simulink model "Copy_of_SbW_can_Add"  (R2023b)
settings: Solver=VariableStepAuto  StartTime=0.0  StopTime=20  RelTol=1e-3
model workspace (MAT data in the model file):
  x = 4
undefined symbols (not defined in the file): canChannel
libraries: simulink x5, canlib x3, canmsglib x2
settings Model: Creator=jcm52  LastModifiedBy=jcm52

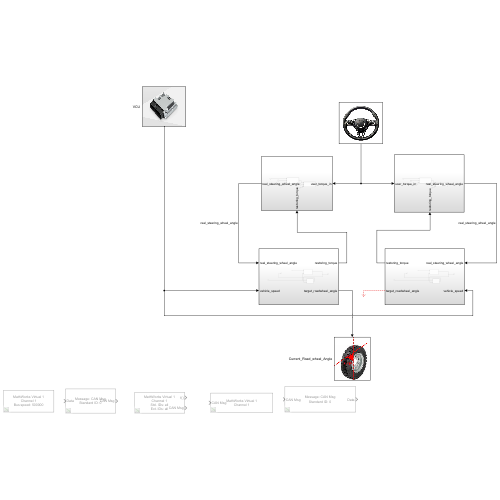
[thumbnail: Simulink's stored preview of the top-level diagram]
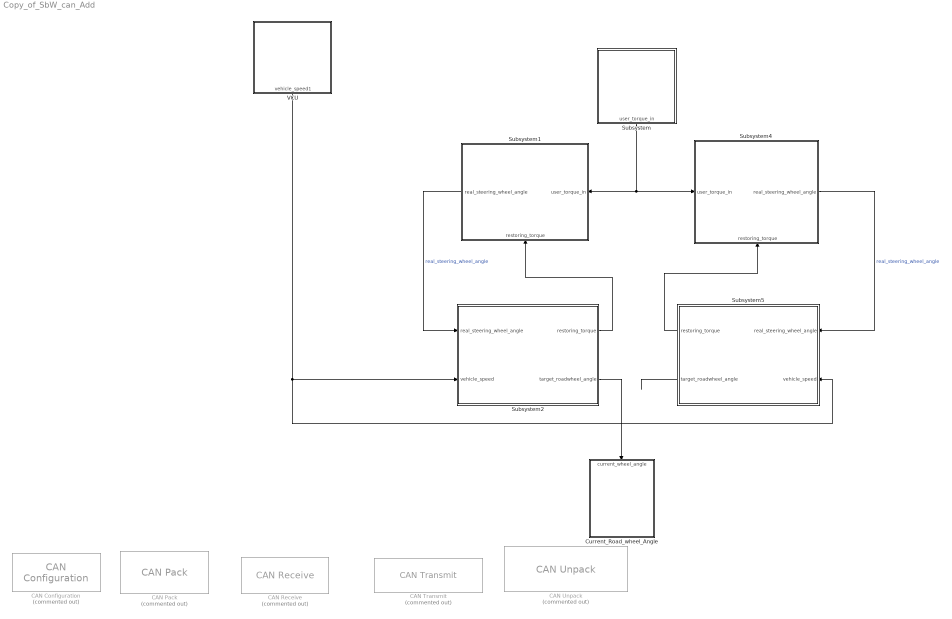
== system Copy_of_SbW_can_Add ==
  CAN Configuration : canlib/CAN Configuration  Commented=on  BlockHandle=2.0012  Device=MathWorks Virtual 1 (Channel 1)  DeviceMenu=MathWorks Virtual 1 (Channel 1)  ObjConstructor=canChannel('MathWorks', 'Virtual 1', 1)  BusSpeed=500000  EnableBitParameters=off  AckMode=Normal
  CAN Pack : canmsglib/CAN Pack  Commented=on  MsgList=(none)  MsgName=CAN Msg  MsgIDType=Standard (11-bit identifier)  MsgIdentifier=0  MsgLength=8  Remote=off  ApplyMinMax=off  BusOutput=off  SignalInfo={}
      settings: LibrarySourceBlock=canlib/CAN Pack  DataFormat=raw data
  CAN Receive : canlib/CAN Receive  Commented=on  BlockHandle=4.0002  Device=MathWorks Virtual 1 (Channel 1)  DeviceMenu=MathWorks Virtual 1 (Channel 1)  ObjConstructor=canChannel('MathWorks', 'Virtual 1', 1)  EnableStandardIDsFilter=off  StdIDsCombo=Allow all  StandardIDs=0  EnableExtendedIDsFilter=off  ExtIDsCombo=Allow all  ExtendedIDs=0  SampleTime=0.01  MsgsPerTimestep=all  InternalFilterUpdateStatus=on  BusOutput=off
  CAN Transmit : canlib/CAN Transmit  Commented=on  BlockHandle=5.0002  Device=MathWorks Virtual 1 (Channel 1)  DeviceMenu=MathWorks Virtual 1 (Channel 1)  ObjConstructor=canChannel('MathWorks', 'Virtual 1', 1)  EnableEventTransmit=off  EnablePeriodicTransmit=off  MessagePeriod=1.000
  CAN Unpack : canmsglib/CAN Unpack  Commented=on  MsgList=(none)  MsgName=CAN Msg  MsgIDType=Standard (11-bit identifier)  MsgIdentifier=0  MsgLength=8  SignalInfo={}  IDPort=off  TimestampPort=off  ErrorPort=off  RemotePort=off  LengthPort=off  StatusPort=off  ApplyMinMax=off
      settings: LibrarySourceBlock=canlib/CAN Unpack  DataFormat=raw data
  Current_Road_wheel_Angle : Subsystem
      mask Display: image('image\road_wheel_angle.JPG');
  Subsystem : Subsystem
      mask Display: image('image\pngtree-car-steering-wheel-png-image_13061877.png');
  Subsystem1 : Subsystem
      settings: PortSchema="{\"entries\":[{\"content\":{\"sides\":[{\"content\":{\"connectorIds\":[\"In1\"]},\"type\":\"ConnectorPlacement.EquallySpacedRectSide\",\"uuid\":\"9f784dfa-5041-4500-abe3-8ca3b2947121\"},{\"content\":{\"connectorIds\":[\"Out1\"],\"side\":\"RIGHT\"},\"type\":\"ConnectorPlacement.EquallySpacedRectSide\",\"uuid\":\"b0f943eb-3587-44b5-9c58-09c6c0469d22\"},{\"content\":{\"connectorIds\":[\"In2\"],\"side\":\"TOP\"},\"type\":\"ConnectorPlacement.EquallySpacedRectSide\",\"uuid\":\"b1f972b4-0000-4041-88f3-3b96e8f3d0bc\"},{\"content\":{\"side\":\"BOTTOM\"},\"type\":\"ConnectorPlacement.EquallySpacedRectSide\",\"uuid\":\"3fad1dd4-0e91-4329-9148-3a998504f86d\"}]},\"type\":\"ConnectorPlacement.EquallySpacedConnector\",\"uuid\":\"65662e9c-02e8-4401-a13c-81033cd1290c\"}],\"packageUris\":[\"http://schema.mathworks.com/mf0/Connector/R2020b\"],\"version\":\"1.0\"}"
  Subsystem2 : Subsystem
  Subsystem4 : Subsystem
      settings: PortSchema="{\"entries\":[{\"content\":{\"sides\":[{\"content\":{\"connectorIds\":[\"In1\"]},\"type\":\"ConnectorPlacement.EquallySpacedRectSide\",\"uuid\":\"9f784dfa-5041-4500-abe3-8ca3b2947121\"},{\"content\":{\"connectorIds\":[\"Out1\"],\"side\":\"RIGHT\"},\"type\":\"ConnectorPlacement.EquallySpacedRectSide\",\"uuid\":\"b0f943eb-3587-44b5-9c58-09c6c0469d22\"},{\"content\":{\"side\":\"TOP\"},\"type\":\"ConnectorPlacement.EquallySpacedRectSide\",\"uuid\":\"b1f972b4-0000-4041-88f3-3b96e8f3d0bc\"},{\"content\":{\"connectorIds\":[\"In2\"],\"side\":\"BOTTOM\"},\"type\":\"ConnectorPlacement.EquallySpacedRectSide\",\"uuid\":\"3fad1dd4-0e91-4329-9148-3a998504f86d\"}]},\"type\":\"ConnectorPlacement.EquallySpacedConnector\",\"uuid\":\"65662e9c-02e8-4401-a13c-81033cd1290c\"}],\"packageUris\":[\"http://schema.mathworks.com/mf0/Connector/R2020b\"],\"version\":\"1.0\"}"
  Subsystem5 : Subsystem
  VCU : Subsystem
      mask Display: image('image\vehicle-control-unit-compare-view-01_teaser.jpg');
  wires:
  Subsystem1/1(real_steering_wheel_angle) -> Subsystem2/1(real_steering_wheel_angle)  "real_steering_wheel_angle"
  Subsystem2/1(restoring_torque) -> Subsystem1/2(restoring_torque)
  Subsystem2/2(target_roadwheel_angle) -> Current_Road_wheel_Angle/1(current_wheel_angle)
  Subsystem/1(user_torque_in) -> Subsystem4/1(user_torque_in), Subsystem1/1(user_torque_in)
  Subsystem4/1(real_steering_wheel_angle) -> Subsystem5/1(real_steering_wheel_angle)  "real_steering_wheel_angle"
  Subsystem5/1(restoring_torque) -> Subsystem4/2(restoring_torque)
  VCU/1(vehicle_speed1) -> Subsystem5/2(vehicle_speed), Subsystem2/2(vehicle_speed)
  Subsystem5/2(target_roadwheel_angle) -> ?

== system Copy_of_SbW_can_Add/Current_Road_wheel_Angle ==
  current_wheel_angle : Inport

== system Copy_of_SbW_can_Add/Subsystem ==
  Bias : Bias  Bias=x  SaturateOnIntegerOverflow=off
  pulse_torque_in2 : DiscretePulseGenerator  PulseType=Time based  Amplitude=2*x  Period=5  PulseWidth=50
      mask Display: image('image\pngtree-car-steering-wheel-png-image_13061877.png');
  user_torque_in : Outport
  wires:
  pulse_torque_in2/1 -> Bias/1  "Torque_in"
  Bias/1 -> user_torque_in/1  "user_torque_in"

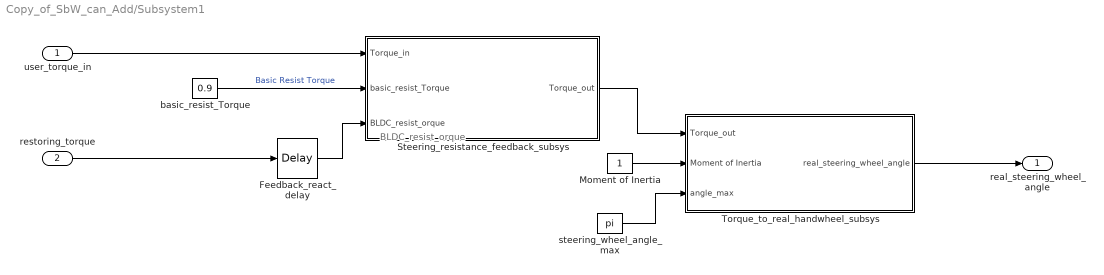
== system Copy_of_SbW_can_Add/Subsystem1 ==
  note: BLDC_resist_orque
  user_torque_in : Inport
  restoring_torque : Inport  Port=2
  Feedback_react_delay : TransportDelay  DelayTime=0.02
  Moment of Inertia : Constant
  Steering_resistance_feedback_subsys : Subsystem
  Torque_to_real_handwheel_subsys : Subsystem
  basic_resist_Torque : Constant  Value=0.9  SampleTime=0.001
  steering_wheel_angle_max : Constant  Value=pi
  real_steering_wheel_angle : Outport
  wires:
  restoring_torque/1 -> Feedback_react_delay/1
  Steering_resistance_feedback_subsys/1(Torque_out) -> Torque_to_real_handwheel_subsys/1(Torque_out)
  steering_wheel_angle_max/1 -> Torque_to_real_handwheel_subsys/3(angle_max)
  Torque_to_real_handwheel_subsys/1(real_steering_wheel_angle) -> real_steering_wheel_angle/1
  Feedback_react_delay/1 -> Steering_resistance_feedback_subsys/3(BLDC_resist_orque)
  Moment of Inertia/1 -> Torque_to_real_handwheel_subsys/2(Moment of Inertia)
  user_torque_in/1 -> Steering_resistance_feedback_subsys/1(Torque_in)
  basic_resist_Torque/1 -> Steering_resistance_feedback_subsys/2(basic_resist_Torque)  "Basic Resist Torque"

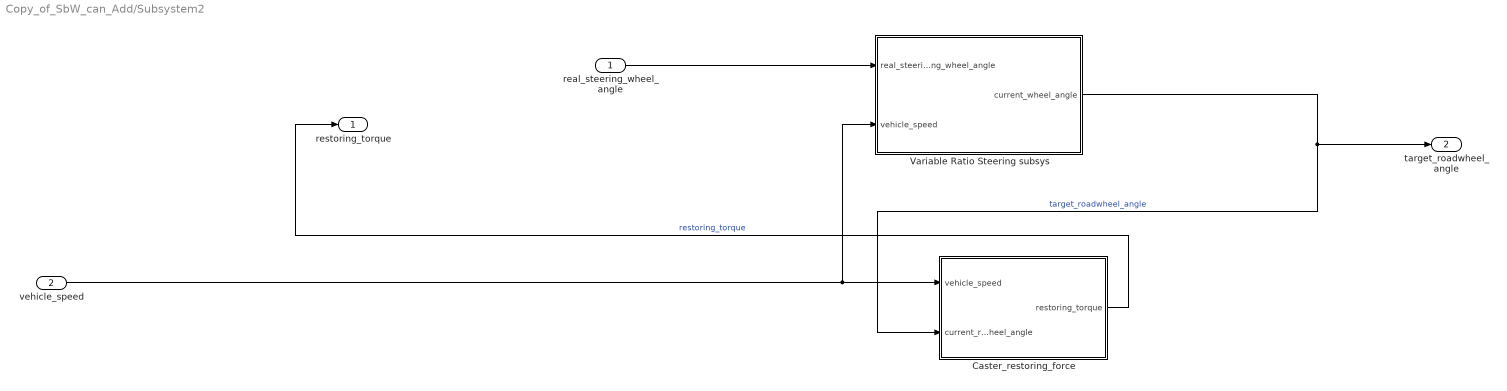
== system Copy_of_SbW_can_Add/Subsystem2 ==
  real_steering_wheel_angle : Inport
  vehicle_speed : Inport  Port=2
  Caster_restoring_force : Subsystem
  Variable Ratio Steering subsys : Subsystem
  restoring_torque : Outport
  target_roadwheel_angle : Outport  Port=2
  wires:
  Variable Ratio Steering subsys/1(current_wheel_angle) -> target_roadwheel_angle/1, Caster_restoring_force/2(current_roadwheel_angle)  "target_roadwheel_angle"
  vehicle_speed/1 -> Variable Ratio Steering subsys/2(vehicle_speed), Caster_restoring_force/1(vehicle_speed)
  Caster_restoring_force/1(restoring_torque) -> restoring_torque/1  "restoring_torque"
  real_steering_wheel_angle/1 -> Variable Ratio Steering subsys/1(real_steering_wheel_angle)

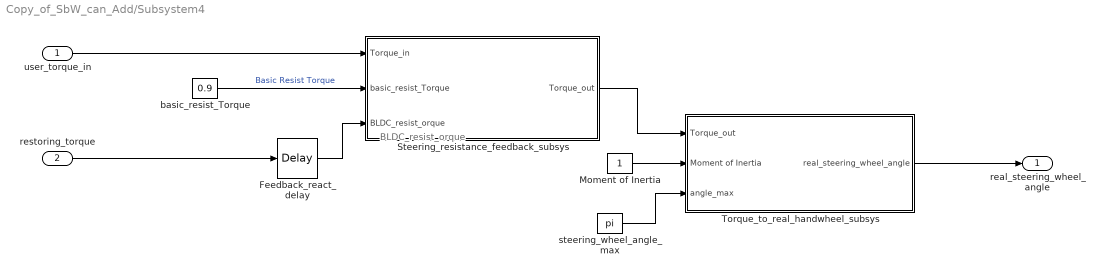
== system Copy_of_SbW_can_Add/Subsystem4 ==
  note: BLDC_resist_orque
  user_torque_in : Inport
  restoring_torque : Inport  Port=2
  Feedback_react_delay : TransportDelay  DelayTime=0.02
  Moment of Inertia : Constant
  Steering_resistance_feedback_subsys : Subsystem
  Torque_to_real_handwheel_subsys : Subsystem
  basic_resist_Torque : Constant  Value=0.9  SampleTime=0.001
  steering_wheel_angle_max : Constant  Value=pi
  real_steering_wheel_angle : Outport
  wires:
  restoring_torque/1 -> Feedback_react_delay/1
  Steering_resistance_feedback_subsys/1(Torque_out) -> Torque_to_real_handwheel_subsys/1(Torque_out)
  steering_wheel_angle_max/1 -> Torque_to_real_handwheel_subsys/3(angle_max)
  Torque_to_real_handwheel_subsys/1(real_steering_wheel_angle) -> real_steering_wheel_angle/1
  Feedback_react_delay/1 -> Steering_resistance_feedback_subsys/3(BLDC_resist_orque)
  Moment of Inertia/1 -> Torque_to_real_handwheel_subsys/2(Moment of Inertia)
  user_torque_in/1 -> Steering_resistance_feedback_subsys/1(Torque_in)
  basic_resist_Torque/1 -> Steering_resistance_feedback_subsys/2(basic_resist_Torque)  "Basic Resist Torque"

== system Copy_of_SbW_can_Add/Subsystem5 ==
  real_steering_wheel_angle : Inport
  vehicle_speed : Inport  Port=2
  Caster_restoring_force : Subsystem
  Variable Ratio Steering subsys : Subsystem
  restoring_torque : Outport
  target_roadwheel_angle : Outport  Port=2
  wires:
  Variable Ratio Steering subsys/1(current_wheel_angle) -> target_roadwheel_angle/1, Caster_restoring_force/2(current_roadwheel_angle)  "target_roadwheel_angle"
  vehicle_speed/1 -> Variable Ratio Steering subsys/2(vehicle_speed), Caster_restoring_force/1(vehicle_speed)
  Caster_restoring_force/1(restoring_torque) -> restoring_torque/1  "restoring_torque"
  real_steering_wheel_angle/1 -> Variable Ratio Steering subsys/1(real_steering_wheel_angle)

== system Copy_of_SbW_can_Add/VCU ==
  Subsystem : Subsystem
      mask Display: image('image\free-icon-speed-1455318.png');
  vehicle_speed1 : Outport
  wires:
  Subsystem/1(vehicle_speed1) -> vehicle_speed1/1

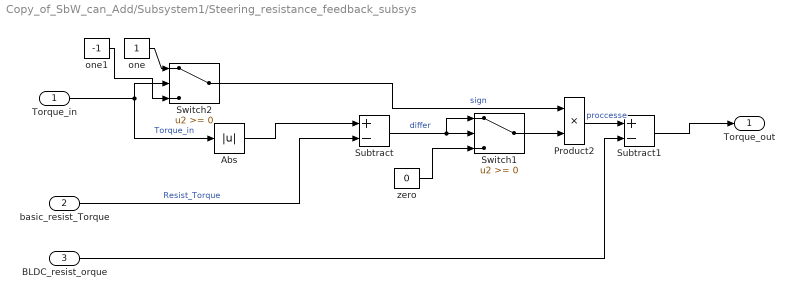
== system Copy_of_SbW_can_Add/Subsystem1/Steering_resistance_feedback_subsys ==
  Torque_in : Inport
  basic_resist_Torque : Inport  Port=2
  BLDC_resist_orque : Inport  Port=3
  Abs : Abs  SaturateOnIntegerOverflow=off
  Product2 : Product
  Subtract : Sum  Inputs=+-
  Subtract1 : Sum  Inputs=+-
  Switch1 : Switch  OutDataTypeStr=double  SaturateOnIntegerOverflow=off  InputSameDT=off
  Switch2 : Switch  OutDataTypeStr=double  SaturateOnIntegerOverflow=off  InputSameDT=off
  one : Constant
  one1 : Constant  Value=-1
  zero : Constant  Value=0
  Torque_out : Outport
  wires:
  Subtract/1 -> Switch1/1, Switch1/2  "differ"
  one/1 -> Switch2/1
  basic_resist_Torque/1 -> Subtract/2  "Resist_Torque"
  zero/1 -> Switch1/3
  Torque_in/1 -> Switch2/2, Abs/1  "Torque_in"
  Switch1/1 -> Product2/2
  Switch2/1 -> Product2/1  "sign"
  Abs/1 -> Subtract/1
  one1/1 -> Switch2/3
  BLDC_resist_orque/1 -> Subtract1/2
  Product2/1 -> Subtract1/1  "proccesse"
  Subtract1/1 -> Torque_out/1

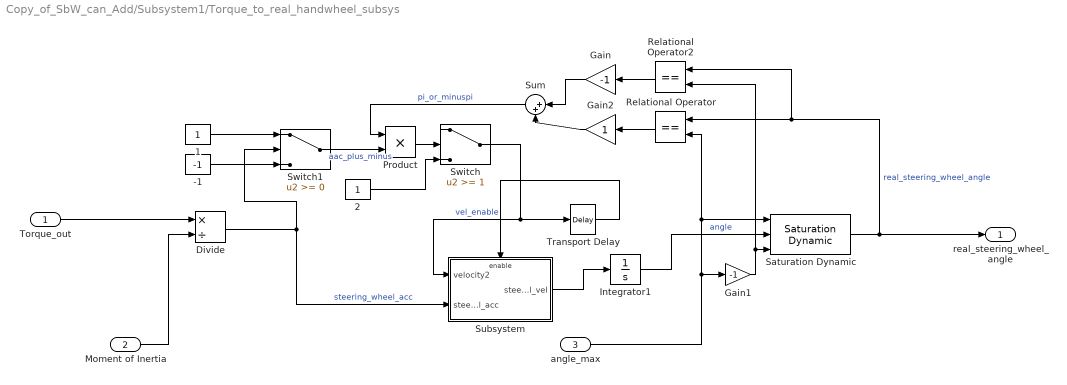
== system Copy_of_SbW_can_Add/Subsystem1/Torque_to_real_handwheel_subsys ==
  Torque_out : Inport
  Moment of Inertia : Inport  Port=2
  angle_max : Inport  Port=3
  -1 : Constant  Value=-1
  1 : Constant
  2 : Constant  OutDataTypeStr=boolean
  Divide : Product  Inputs=*/
  Gain : Gain  Gain=-1
  Gain1 : Gain  Gain=-1
  Gain2 : Gain
  Integrator1 : Integrator
  Product : Product
  Relational Operator : RelationalOperator  Operator===  OutDataTypeStr=boolean  RndMeth=Simplest  InputSameDT=off
  Relational Operator2 : RelationalOperator  Operator===  OutDataTypeStr=boolean  RndMeth=Simplest  InputSameDT=off
  Saturation Dynamic : simulink/Discontinuities/Saturation Dynamic  OutMin=[]  OutMax=[]  OutDataTypeStr=double  OutDataType=fixdt(1, 16)  OutScaling=2^-10  DoSatur=off
  Subsystem : Subsystem
  Sum : Sum  Inputs=|++
  Switch : Switch  Threshold=1  OutDataTypeStr=double  SaturateOnIntegerOverflow=off  InputSameDT=off
  Switch1 : Switch  SaturateOnIntegerOverflow=off  InputSameDT=off
  Transport Delay : TransportDelay  DelayTime=0.001
  real_steering_wheel_angle : Outport
  wires:
  Saturation Dynamic/1 -> Relational Operator2/1, Relational Operator/1, real_steering_wheel_angle/1  "real_steering_wheel_angle"
  Torque_out/1 -> Divide/1
  Integrator1/1 -> Saturation Dynamic/2  "angle"
  angle_max/1 -> Relational Operator/2, Saturation Dynamic/1, Gain1/1
  Gain1/1 -> Relational Operator2/2, Saturation Dynamic/3
  Moment of Inertia/1 -> Divide/2
  Divide/1 -> Switch1/2, Subsystem/2(steering_wheel_acc)  "steering_wheel_acc"
  Subsystem/1(steering_wheel_vel) -> Integrator1/1
  Switch/1 -> Subsystem/1(velocity2), Transport Delay/1  "vel_enable"
  Sum/1 -> Product/1  "pi_or_minuspi"
  -1/1 -> Switch1/3
  1/1 -> Switch1/1
  Switch1/1 -> Product/2  "aac_plus_minus"
  Relational Operator2/1 -> Gain/1
  Relational Operator/1 -> Gain2/1
  Gain/1 -> Sum/1
  Product/1 -> Switch/2
  2/1 -> Switch/3
  Gain2/1 -> Sum/2
  Transport Delay/1 -> Subsystem/Enable

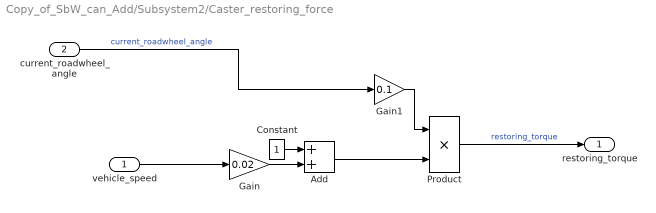
== system Copy_of_SbW_can_Add/Subsystem2/Caster_restoring_force ==
  vehicle_speed : Inport
  current_roadwheel_angle : Inport  Port=2
  Add : Sum
  Constant : Constant
  Gain : Gain  Gain=0.02
  Gain1 : Gain  Gain=0.1
  Product : Product
  restoring_torque : Outport
  wires:
  vehicle_speed/1 -> Gain/1
  Gain/1 -> Add/2
  Constant/1 -> Add/1
  Add/1 -> Product/2
  Gain1/1 -> Product/1
  Product/1 -> restoring_torque/1  "restoring_torque"
  current_roadwheel_angle/1 -> Gain1/1  "current_roadwheel_angle"

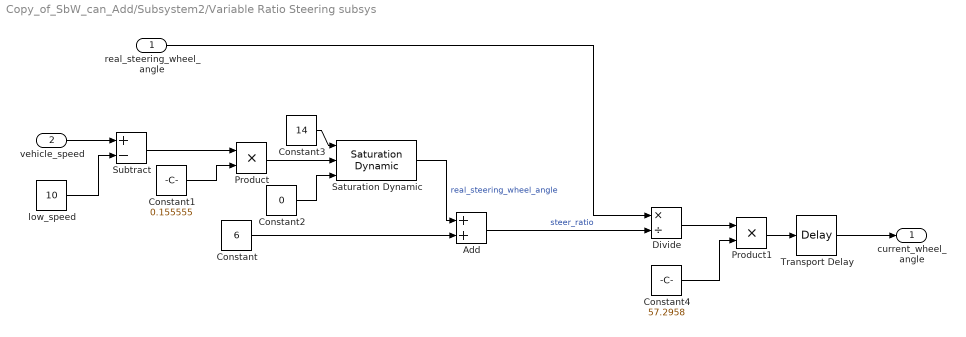
== system Copy_of_SbW_can_Add/Subsystem2/Variable Ratio Steering subsys ==
  real_steering_wheel_angle : Inport
  vehicle_speed : Inport  Port=2
  Add : Sum
  Constant : Constant  Value=6
  Constant1 : Constant  Value=0.155555
  Constant2 : Constant  Value=0
  Constant3 : Constant  Value=14
  Constant4 : Constant  Value=57.2958
  Divide : Product  Inputs=*/
  Product : Product
  Product1 : Product
  Saturation Dynamic : simulink/Discontinuities/Saturation Dynamic  OutMin=[]  OutMax=[]  OutDataTypeStr=double  OutDataType=fixdt(1, 16)  OutScaling=2^-10  DoSatur=off
  Subtract : Sum  Inputs=+-
  Transport Delay : TransportDelay  DelayTime=0.1
  low_speed : Constant  Value=10
  current_wheel_angle : Outport
  wires:
  vehicle_speed/1 -> Subtract/1
  low_speed/1 -> Subtract/2
  Subtract/1 -> Product/1
  Constant1/1 -> Product/2
  Constant/1 -> Add/2
  Product/1 -> Saturation Dynamic/2
  Constant2/1 -> Saturation Dynamic/3
  Constant3/1 -> Saturation Dynamic/1
  Saturation Dynamic/1 -> Add/1  "real_steering_wheel_angle"
  Add/1 -> Divide/2  "steer_ratio"
  real_steering_wheel_angle/1 -> Divide/1
  Divide/1 -> Product1/1
  Constant4/1 -> Product1/2
  Product1/1 -> Transport Delay/1
  Transport Delay/1 -> current_wheel_angle/1

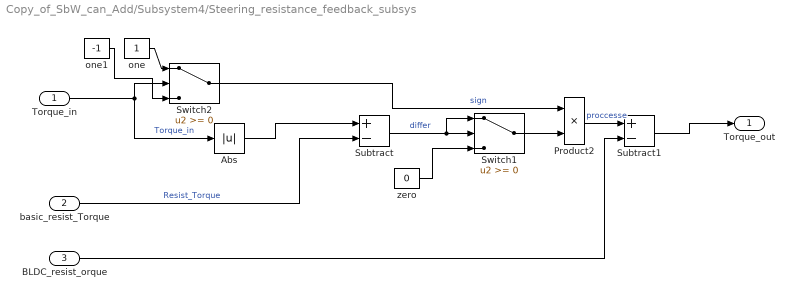
== system Copy_of_SbW_can_Add/Subsystem4/Steering_resistance_feedback_subsys ==
  Torque_in : Inport
  basic_resist_Torque : Inport  Port=2
  BLDC_resist_orque : Inport  Port=3
  Abs : Abs  SaturateOnIntegerOverflow=off
  Product2 : Product
  Subtract : Sum  Inputs=+-
  Subtract1 : Sum  Inputs=+-
  Switch1 : Switch  OutDataTypeStr=double  SaturateOnIntegerOverflow=off  InputSameDT=off
  Switch2 : Switch  OutDataTypeStr=double  SaturateOnIntegerOverflow=off  InputSameDT=off
  one : Constant
  one1 : Constant  Value=-1
  zero : Constant  Value=0
  Torque_out : Outport
  wires:
  Subtract/1 -> Switch1/1, Switch1/2  "differ"
  one/1 -> Switch2/1
  basic_resist_Torque/1 -> Subtract/2  "Resist_Torque"
  zero/1 -> Switch1/3
  Torque_in/1 -> Switch2/2, Abs/1  "Torque_in"
  Switch1/1 -> Product2/2
  Switch2/1 -> Product2/1  "sign"
  Abs/1 -> Subtract/1
  one1/1 -> Switch2/3
  BLDC_resist_orque/1 -> Subtract1/2
  Product2/1 -> Subtract1/1  "proccesse"
  Subtract1/1 -> Torque_out/1

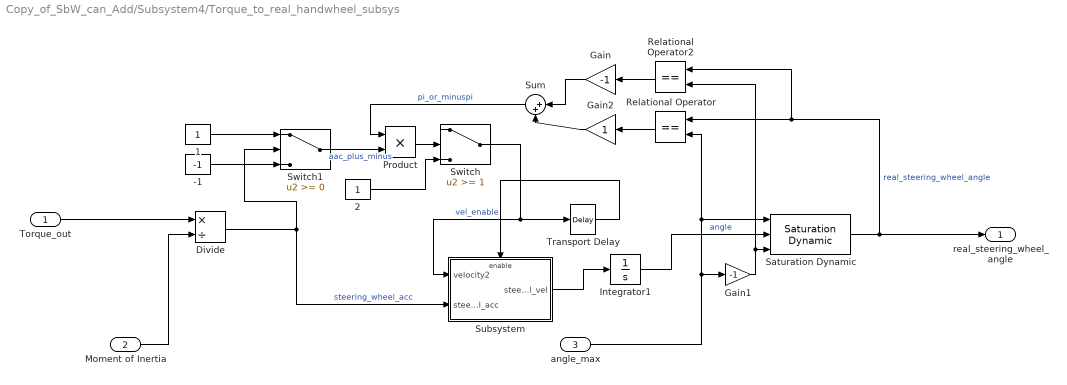
== system Copy_of_SbW_can_Add/Subsystem4/Torque_to_real_handwheel_subsys ==
  Torque_out : Inport
  Moment of Inertia : Inport  Port=2
  angle_max : Inport  Port=3
  -1 : Constant  Value=-1
  1 : Constant
  2 : Constant  OutDataTypeStr=boolean
  Divide : Product  Inputs=*/
  Gain : Gain  Gain=-1
  Gain1 : Gain  Gain=-1
  Gain2 : Gain
  Integrator1 : Integrator
  Product : Product
  Relational Operator : RelationalOperator  Operator===  OutDataTypeStr=boolean  RndMeth=Simplest  InputSameDT=off
  Relational Operator2 : RelationalOperator  Operator===  OutDataTypeStr=boolean  RndMeth=Simplest  InputSameDT=off
  Saturation Dynamic : simulink/Discontinuities/Saturation Dynamic  OutMin=[]  OutMax=[]  OutDataTypeStr=double  OutDataType=fixdt(1, 16)  OutScaling=2^-10  DoSatur=off
  Subsystem : Subsystem
  Sum : Sum  Inputs=|++
  Switch : Switch  Threshold=1  OutDataTypeStr=double  SaturateOnIntegerOverflow=off  InputSameDT=off
  Switch1 : Switch  SaturateOnIntegerOverflow=off  InputSameDT=off
  Transport Delay : TransportDelay  DelayTime=0.001
  real_steering_wheel_angle : Outport
  wires:
  Saturation Dynamic/1 -> Relational Operator2/1, Relational Operator/1, real_steering_wheel_angle/1  "real_steering_wheel_angle"
  Torque_out/1 -> Divide/1
  Integrator1/1 -> Saturation Dynamic/2  "angle"
  angle_max/1 -> Relational Operator/2, Saturation Dynamic/1, Gain1/1
  Gain1/1 -> Relational Operator2/2, Saturation Dynamic/3
  Moment of Inertia/1 -> Divide/2
  Divide/1 -> Switch1/2, Subsystem/2(steering_wheel_acc)  "steering_wheel_acc"
  Subsystem/1(steering_wheel_vel) -> Integrator1/1
  Switch/1 -> Subsystem/1(velocity2), Transport Delay/1  "vel_enable"
  Sum/1 -> Product/1  "pi_or_minuspi"
  -1/1 -> Switch1/3
  1/1 -> Switch1/1
  Switch1/1 -> Product/2  "aac_plus_minus"
  Relational Operator2/1 -> Gain/1
  Relational Operator/1 -> Gain2/1
  Gain/1 -> Sum/1
  Product/1 -> Switch/2
  2/1 -> Switch/3
  Gain2/1 -> Sum/2
  Transport Delay/1 -> Subsystem/Enable

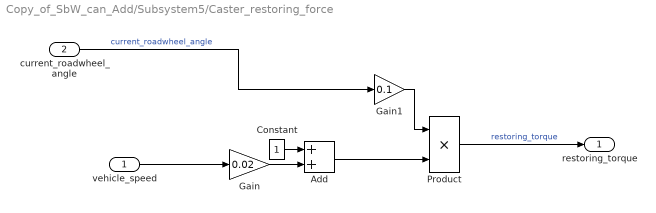
== system Copy_of_SbW_can_Add/Subsystem5/Caster_restoring_force ==
  vehicle_speed : Inport
  current_roadwheel_angle : Inport  Port=2
  Add : Sum
  Constant : Constant
  Gain : Gain  Gain=0.02
  Gain1 : Gain  Gain=0.1
  Product : Product
  restoring_torque : Outport
  wires:
  vehicle_speed/1 -> Gain/1
  Gain/1 -> Add/2
  Constant/1 -> Add/1
  Add/1 -> Product/2
  Gain1/1 -> Product/1
  Product/1 -> restoring_torque/1  "restoring_torque"
  current_roadwheel_angle/1 -> Gain1/1  "current_roadwheel_angle"

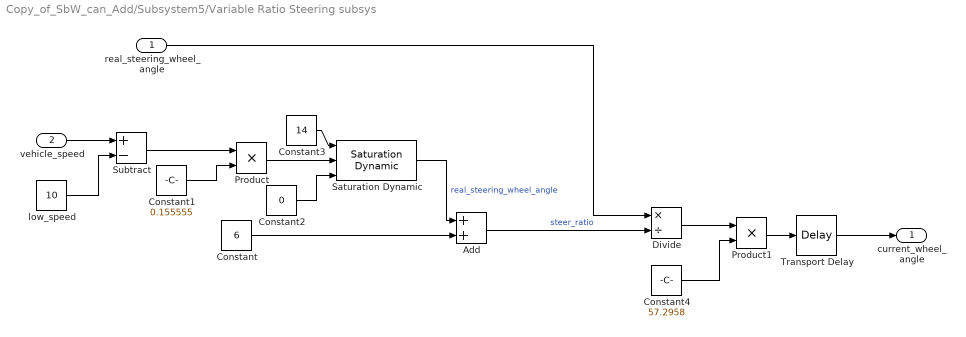
== system Copy_of_SbW_can_Add/Subsystem5/Variable Ratio Steering subsys ==
  real_steering_wheel_angle : Inport
  vehicle_speed : Inport  Port=2
  Add : Sum
  Constant : Constant  Value=6
  Constant1 : Constant  Value=0.155555
  Constant2 : Constant  Value=0
  Constant3 : Constant  Value=14
  Constant4 : Constant  Value=57.2958
  Divide : Product  Inputs=*/
  Product : Product
  Product1 : Product
  Saturation Dynamic : simulink/Discontinuities/Saturation Dynamic  OutMin=[]  OutMax=[]  OutDataTypeStr=double  OutDataType=fixdt(1, 16)  OutScaling=2^-10  DoSatur=off
  Subtract : Sum  Inputs=+-
  Transport Delay : TransportDelay  DelayTime=0.1
  low_speed : Constant  Value=10
  current_wheel_angle : Outport
  wires:
  vehicle_speed/1 -> Subtract/1
  low_speed/1 -> Subtract/2
  Subtract/1 -> Product/1
  Constant1/1 -> Product/2
  Constant/1 -> Add/2
  Product/1 -> Saturation Dynamic/2
  Constant2/1 -> Saturation Dynamic/3
  Constant3/1 -> Saturation Dynamic/1
  Saturation Dynamic/1 -> Add/1  "real_steering_wheel_angle"
  Add/1 -> Divide/2  "steer_ratio"
  real_steering_wheel_angle/1 -> Divide/1
  Divide/1 -> Product1/1
  Constant4/1 -> Product1/2
  Product1/1 -> Transport Delay/1
  Transport Delay/1 -> current_wheel_angle/1

== system Copy_of_SbW_can_Add/VCU/Subsystem ==
  vehicle_speed : simulink/Sources/Repeating Sequence  rep_seq_t=[0 50 100]  rep_seq_y=[0 200 0]
  vehicle_speed1 : Outport
  wires:
  vehicle_speed/1 -> vehicle_speed1/1  "vehicle_speed"

== system Copy_of_SbW_can_Add/Subsystem1/Torque_to_real_handwheel_subsys/Subsystem ==
  velocity2 : Inport
  steering_wheel_acc : Inport  Port=2
  Enable : EnablePort  StatesWhenEnabling=reset
  Integrator : Integrator  ExternalReset=either
  steering_wheel_vel : Outport
  wires:
  Integrator/1 -> steering_wheel_vel/1  "steering_wheel_vel"
  velocity2/1 -> Integrator/2
  steering_wheel_acc/1 -> Integrator/1

== system Copy_of_SbW_can_Add/Subsystem4/Torque_to_real_handwheel_subsys/Subsystem ==
  velocity2 : Inport
  steering_wheel_acc : Inport  Port=2
  Enable : EnablePort  StatesWhenEnabling=reset
  Integrator : Integrator  ExternalReset=either
  steering_wheel_vel : Outport
  wires:
  Integrator/1 -> steering_wheel_vel/1  "steering_wheel_vel"
  velocity2/1 -> Integrator/2
  steering_wheel_acc/1 -> Integrator/1
